simulink model "linearization"  (Simulink 8.7)
settings: Solver=VariableStepAuto  StartTime=0.0  StopTime=10.0  RelTol=1e-3
undefined symbols (not defined in the file or in its folder): CONFIG, DiscIntNeverNeededParam, gain, reg, ROBOT_DOF, ROBOT_DOF_FOR_SIMULINK, WBT_robotName
libraries: WBToolboxLibrary x42
settings Model: Creator=gnava  LastModifiedBy=gnava
settings DataIOCC: LimitDataPoints=off  SaveFormat=Dataset
settings DebuggingCC: UnderspecifiedInitializationDetection=Simplified  MergeDetectMultiDrivingBlocksExec=error
settings HardwareCC: ProdBitPerPointer=64  ProdLargestAtomicFloat=Float  ProdIntDivRoundTo=Zero  ProdEndianess=LittleEndian  ProdWordSize=64  ProdHWDeviceType=Intel->x86-64 (Windows64)
settings ModelReferenceCC: PropagateSignalLabelsOutOfModel=on
settings ConfigComp: CovModelRefEnable=off

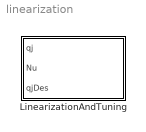
== system linearization ==
  LinearizationAndTuning : Subsystem

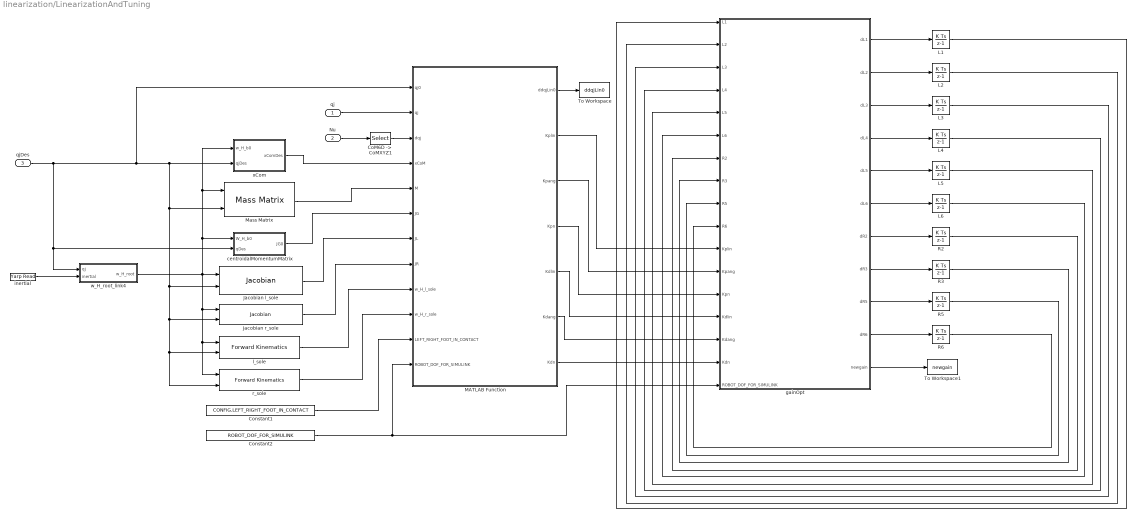
== system linearization/LinearizationAndTuning ==
  qj : Inport
  Nu : Inport  Port=2
  qjDes : Inport  Port=3
  "CoM6D ->  CoMXYZ1" : Selector  InputPortWidth=6+ROBOT_DOF  IndexOptions=Index vector (dialog)  Indices=[7:6+ROBOT_DOF]  OutputSizes=1
  Constant1 : Constant  Value=CONFIG.LEFT_RIGHT_FOOT_IN_CONTACT
  Constant2 : Constant  Value=ROBOT_DOF_FOR_SIMULINK
  Jacobian l_sole : WBToolboxLibrary/wholeBodyModel/Jacobians/Jacobian  frameName='l_sole'  robotName=WBT_robotName  localName=WBT_modelName  wbiFile=WBT_wbiFilename  wbiList=WBT_wbiList
  Jacobian r_sole : WBToolboxLibrary/wholeBodyModel/Jacobians/Jacobian  frameName='r_sole'  robotName=WBT_robotName  localName=WBT_modelName  wbiFile=WBT_wbiFilename  wbiList=WBT_wbiList
  L1 : DiscreteIntegrator  InitialCondition=gain.CI1  InitialConditionSetting=State (most efficient)  SampleTime=CONFIG.Ts  ICPrevOutput=DiscIntNeverNeededParam  ICPrevScaledInput=DiscIntNeverNeededParam
  L2 : DiscreteIntegrator  InitialCondition=gain.CI2  InitialConditionSetting=State (most efficient)  SampleTime=CONFIG.Ts  ICPrevOutput=DiscIntNeverNeededParam  ICPrevScaledInput=DiscIntNeverNeededParam
  L3 : DiscreteIntegrator  InitialCondition=gain.CI3  InitialConditionSetting=State (most efficient)  SampleTime=CONFIG.Ts  ICPrevOutput=DiscIntNeverNeededParam  ICPrevScaledInput=DiscIntNeverNeededParam
  L4 : DiscreteIntegrator  InitialCondition=gain.CI4  InitialConditionSetting=State (most efficient)  SampleTime=CONFIG.Ts  ICPrevOutput=DiscIntNeverNeededParam  ICPrevScaledInput=DiscIntNeverNeededParam
  L5 : DiscreteIntegrator  InitialCondition=gain.CI5  InitialConditionSetting=State (most efficient)  SampleTime=CONFIG.Ts  ICPrevOutput=DiscIntNeverNeededParam  ICPrevScaledInput=DiscIntNeverNeededParam
  L6 : DiscreteIntegrator  InitialCondition=gain.CI6  InitialConditionSetting=State (most efficient)  SampleTime=CONFIG.Ts  ICPrevOutput=DiscIntNeverNeededParam  ICPrevScaledInput=DiscIntNeverNeededParam
  MATLAB Function : MATLAB Function  TreatAsAtomicUnit=on
  Mass Matrix : WBToolboxLibrary/wholeBodyModel/Dynamics/Mass Matrix  robotName=WBT_robotName  localName=WBT_modelName  wbiFile=WBT_wbiFilename  wbiList=WBT_wbiList
  R2 : DiscreteIntegrator  InitialCondition=eye(3)  InitialConditionSetting=State (most efficient)  SampleTime=CONFIG.Ts  ICPrevOutput=DiscIntNeverNeededParam  ICPrevScaledInput=DiscIntNeverNeededParam
  R3 : DiscreteIntegrator  InitialCondition=eye(ROBOT_DOF)  InitialConditionSetting=State (most efficient)  SampleTime=CONFIG.Ts  ICPrevOutput=DiscIntNeverNeededParam  ICPrevScaledInput=DiscIntNeverNeededParam
  R5 : DiscreteIntegrator  InitialCondition=eye(3)  InitialConditionSetting=State (most efficient)  SampleTime=CONFIG.Ts  ICPrevOutput=DiscIntNeverNeededParam  ICPrevScaledInput=DiscIntNeverNeededParam
  R6 : DiscreteIntegrator  InitialCondition=eye(ROBOT_DOF)  InitialConditionSetting=State (most efficient)  SampleTime=CONFIG.Ts  ICPrevOutput=DiscIntNeverNeededParam  ICPrevScaledInput=DiscIntNeverNeededParam
  To Workspace : ToWorkspace  VariableName=ddqjLin0  SaveFormat=Structure With Time  SampleTime=-1
  To Workspace1 : ToWorkspace  VariableName=newgain  SaveFormat=Structure With Time  SampleTime=-1
  centroidalMomentumMatrix : Subsystem
  gainOpt : MATLAB Function  TreatAsAtomicUnit=on
  inertial : WBToolboxLibrary/Utilities/Yarp Read  portName=PORTS.IMU  signalSize=12  blocking=off  timestamp=off  autoconnect=on  errorOnConnection=on
  l_sole : WBToolboxLibrary/wholeBodyModel/Kinematics/Forward Kinematics  frameName='l_sole'  robotName=WBT_robotName  localName=WBT_modelName  wbiFile=WBT_wbiFilename  wbiList=WBT_wbiList
  r_sole : WBToolboxLibrary/wholeBodyModel/Kinematics/Forward Kinematics  frameName='r_sole'  robotName=WBT_robotName  localName=WBT_modelName  wbiFile=WBT_wbiFilename  wbiList=WBT_wbiList
  w_H_root_link4 : Subsystem  mask{link_name='l_sole'}
      mask prompts: link_name "link name"
      mask help:
      | This block evaluates the homogeneous transformation between the world and the root link, i.e. ^wH_b. It assumes that the link specified by the variable 'link_name' has a constant position
      | w.r.t. an inertial frame, but it can rotate arbitrarily. This rotation is retrived from the IMU sensor.
      mask Display:
      | str = strrep(link_name, '_','\_');
      | port_label('output',1,['{}^{',str '}H_{root}'],'texmode','on')
      | clear str;
      | 
      | port_label('input',1,'q_j','texmode','on')
      | 
      | port_label('input',2,'inertial','texmode','on')
  xCom : Subsystem
  wires:
  w_H_root_link4/1(w_H_root) -> xCom/1(w_H_b0), Mass Matrix/1, centroidalMomentumMatrix/1(W_H_b0), Jacobian l_sole/1, Jacobian r_sole/1, l_sole/1, r_sole/1
  inertial/1 -> w_H_root_link4/2(inertial)
  qjDes/1 -> Mass Matrix/2, Jacobian l_sole/2, Jacobian r_sole/2, l_sole/2, r_sole/2, xCom/2(qjDes), MATLAB Function/1(qj0), w_H_root_link4/1(qj), centroidalMomentumMatrix/2(qDes)
  xCom/1(xComDes) -> MATLAB Function/4(xCoM)
  Mass Matrix/1 -> MATLAB Function/5(M)
  Constant1/1 -> MATLAB Function/11(LEFT_RIGHT_FOOT_IN_CONTACT)
  Jacobian l_sole/1 -> MATLAB Function/7(JL)
  Jacobian r_sole/1 -> MATLAB Function/8(JR)
  l_sole/1 -> MATLAB Function/9(w_H_l_sole)
  r_sole/1 -> MATLAB Function/10(w_H_r_sole)
  centroidalMomentumMatrix/1(JG0) -> MATLAB Function/6(JG)
  Nu/1 -> "CoM6D ->  CoMXYZ1"/1
  qj/1 -> MATLAB Function/2(qj)
  "CoM6D ->  CoMXYZ1"/1 -> MATLAB Function/3(dqj)
  MATLAB Function/1(ddqjLin0) -> To Workspace/1
  Constant2/1 -> gainOpt/17(ROBOT_DOF_FOR_SIMULINK), MATLAB Function/12(ROBOT_DOF_FOR_SIMULINK)
  MATLAB Function/7(Kdn) -> gainOpt/16(Kdn)
  MATLAB Function/6(Kdang) -> gainOpt/15(Kdang)
  MATLAB Function/5(Kdlin) -> gainOpt/14(Kdlin)
  MATLAB Function/4(Kpn) -> gainOpt/13(Kpn)
  MATLAB Function/3(Kpang) -> gainOpt/12(Kpang)
  MATLAB Function/2(Kplin) -> gainOpt/11(Kplin)
  gainOpt/11(newgain) -> To Workspace1/1
  gainOpt/1(dL1) -> L1/1
  gainOpt/2(dL2) -> L2/1
  gainOpt/3(dL3) -> L3/1
  gainOpt/4(dL4) -> L4/1
  gainOpt/5(dL5) -> L5/1
  gainOpt/6(dL6) -> L6/1
  gainOpt/7(dR2) -> R2/1
  gainOpt/8(dR3) -> R3/1
  gainOpt/9(dR5) -> R5/1
  gainOpt/10(dR6) -> R6/1
  L1/1 -> gainOpt/1(L1)
  L2/1 -> gainOpt/2(L2)
  L3/1 -> gainOpt/3(L3)
  L4/1 -> gainOpt/4(L4)
  L5/1 -> gainOpt/5(L5)
  L6/1 -> gainOpt/6(L6)
  R2/1 -> gainOpt/7(R2)
  R3/1 -> gainOpt/8(R3)
  R5/1 -> gainOpt/9(R5)
  R6/1 -> gainOpt/10(R6)

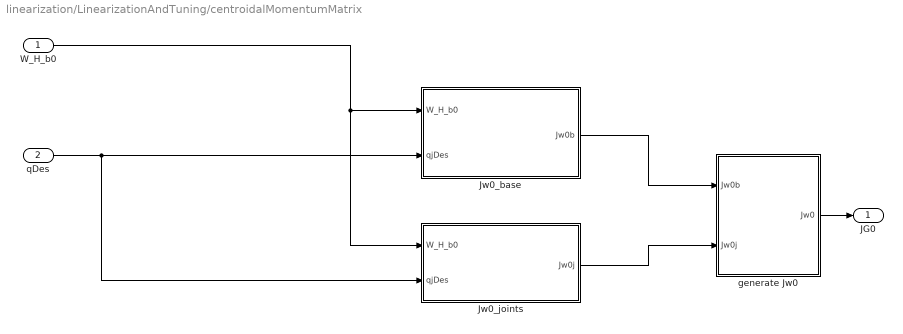
== system linearization/LinearizationAndTuning/centroidalMomentumMatrix ==
  W_H_b0 : Inport
  qDes : Inport  Port=2
  Jw0_base : Subsystem
  Jw0_joints : Subsystem
  generate Jw0 : MATLAB Function  TreatAsAtomicUnit=on
  JG0 : Outport
  wires:
  generate Jw0/1(Jw0) -> JG0/1
  W_H_b0/1 -> Jw0_joints/1(W_H_b0), Jw0_base/1(W_H_b0)
  qDes/1 -> Jw0_base/2(qjDes), Jw0_joints/2(qjDes)
  Jw0_base/1(Jw0b) -> generate Jw0/1(Jw0b)
  Jw0_joints/1(Jw0j) -> generate Jw0/2(Jw0j)

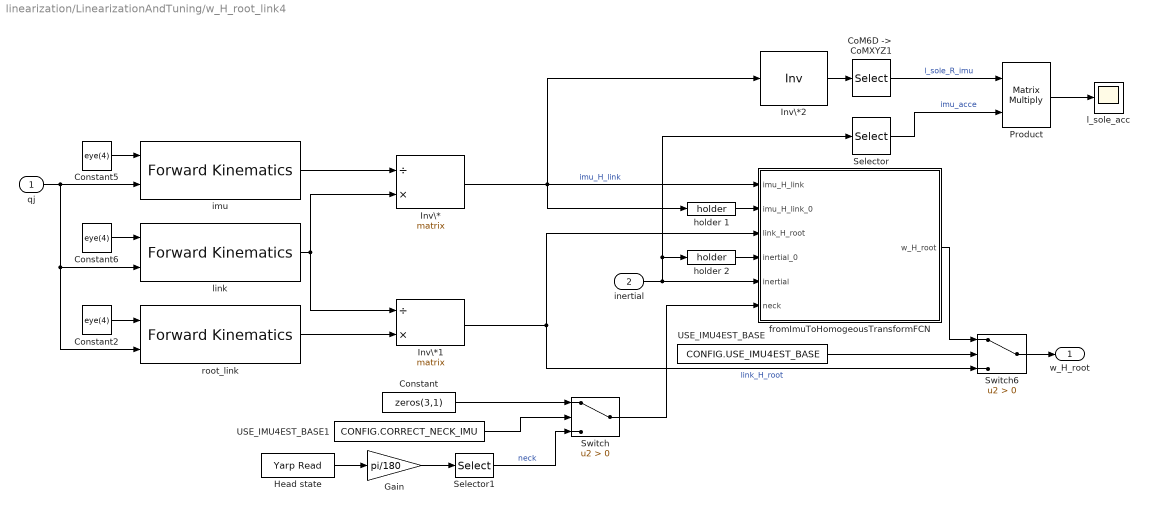
== system linearization/LinearizationAndTuning/w_H_root_link4 ==
  qj : Inport
  inertial : Inport  Port=2
  "CoM6D ->  CoMXYZ1" : Selector  NumberOfDimensions=2  InputPortWidth=7  IndexOptions=Index vector (dialog),Index vector (dialog)  Indices=[1 2 3],[1 2 3]  OutputSizes=1,1
  Constant : Constant  Value=zeros(3,1)
  Constant2 : Constant  Value=eye(4)
  Constant5 : Constant  Value=eye(4)
  Constant6 : Constant  Value=eye(4)
  Gain : Gain  Gain=pi/180
  Head state : WBToolboxLibrary/Utilities/Yarp Read  portName=[WBT_robotName, '/head/state:o']  signalSize=6  blocking=off  timestamp=off  autoconnect=on  errorOnConnection=off
  Inv\* : Product  Inputs=/*  Multiplication=Matrix(*)
  Inv\*1 : Product  Inputs=/*  Multiplication=Matrix(*)
  Inv\*2 : Product  Inputs=/  Multiplication=Matrix(*)
  Product : Product  Multiplication=Matrix(*)
  Selector : Selector  InputPortWidth=12  IndexOptions=Index vector (dialog)  Indices=[4 5 6 ]  OutputSizes=1
  Selector1 : Selector  InputPortWidth=6  IndexOptions=Index vector (dialog)  Indices=[1:3]  OutputSizes=1
  Switch : Switch  Criteria=u2 > Threshold
  Switch6 : Switch  Criteria=u2 > Threshold
  USE_IMU4EST_BASE : Constant  Value=CONFIG.USE_IMU4EST_BASE
  USE_IMU4EST_BASE1 : Constant  Value=CONFIG.CORRECT_NECK_IMU
  fromImuToHomogeousTransformFCN : MATLAB Function  TreatAsAtomicUnit=on
  holder 1 : WBToolboxLibrary/Utilities/holder 
  holder 2 : WBToolboxLibrary/Utilities/holder 
  imu : WBToolboxLibrary/wholeBodyModel/Kinematics/Forward Kinematics  frameName='imu_frame'  robotName=WBT_robotName  localName=WBT_modelName  wbiFile=WBT_wbiFilename  wbiList=WBT_wbiList
  l_sole_acc : Scope
  link : WBToolboxLibrary/wholeBodyModel/Kinematics/Forward Kinematics  frameName=link_name  robotName=WBT_robotName  localName=WBT_modelName  wbiFile=WBT_wbiFilename  wbiList=WBT_wbiList
  root_link : WBToolboxLibrary/wholeBodyModel/Kinematics/Forward Kinematics  frameName='root_link'  robotName=WBT_robotName  localName=WBT_modelName  wbiFile=WBT_wbiFilename  wbiList=WBT_wbiList
  w_H_root : Outport
  wires:
  Constant5/1 -> imu/1
  Inv\*/1 -> Inv\*2/1, holder 1/1, fromImuToHomogeousTransformFCN/1(imu_H_link)  "imu_H_link"
  imu/1 -> Inv\*/1
  Constant6/1 -> link/1
  Inv\*1/1 -> Switch6/3, fromImuToHomogeousTransformFCN/3(link_H_root)  "link_H_root"
  link/1 -> Inv\*/2, Inv\*1/1
  inertial/1 -> Selector/1, holder 2/1, fromImuToHomogeousTransformFCN/5(inertial)
  Switch6/1 -> w_H_root/1
  USE_IMU4EST_BASE/1 -> Switch6/2
  fromImuToHomogeousTransformFCN/1(w_H_root) -> Switch6/1
  Constant2/1 -> root_link/1
  qj/1 -> root_link/2, link/2, imu/2
  root_link/1 -> Inv\*1/2
  holder 1/1 -> fromImuToHomogeousTransformFCN/2(imu_H_link_0)
  holder 2/1 -> fromImuToHomogeousTransformFCN/4(inertial_0)
  Inv\*2/1 -> "CoM6D ->  CoMXYZ1"/1
  "CoM6D ->  CoMXYZ1"/1 -> Product/1  "l_sole_R_imu"
  Selector/1 -> Product/2  "imu_acce"
  Product/1 -> l_sole_acc/1
  Head state/1 -> Gain/1
  Selector1/1 -> Switch/3  "neck"
  Constant/1 -> Switch/1
  USE_IMU4EST_BASE1/1 -> Switch/2
  Switch/1 -> fromImuToHomogeousTransformFCN/6(neck)
  Gain/1 -> Selector1/1

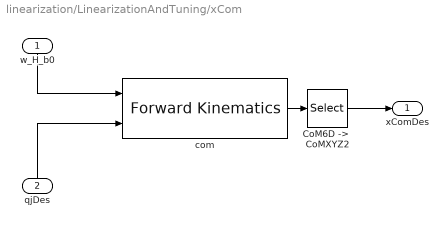
== system linearization/LinearizationAndTuning/xCom ==
  w_H_b0 : Inport
  qjDes : Inport  Port=2
  "CoM6D ->  CoMXYZ2" : Selector  NumberOfDimensions=2  InputPortWidth=7  IndexOptions=Index vector (dialog),Index vector (dialog)  Indices=[1 2 3],[4]  OutputSizes=1,1
  com : WBToolboxLibrary/wholeBodyModel/Kinematics/Forward Kinematics  frameName='com'  robotName=WBT_robotName  localName=WBT_modelName  wbiFile=WBT_wbiFilename  wbiList=WBT_wbiList
  xComDes : Outport
  wires:
  qjDes/1 -> com/2
  "CoM6D ->  CoMXYZ2"/1 -> xComDes/1
  com/1 -> "CoM6D ->  CoMXYZ2"/1
  w_H_b0/1 -> com/1

== system linearization/LinearizationAndTuning/centroidalMomentumMatrix/Jw0_base ==
  W_H_b0 : Inport
  qjDes : Inport  Port=2
  Generate_Jw0base : Subsystem
  Jw0b : Outport
  wires:
  Generate_Jw0base/1(Jw0b) -> Jw0b/1
  qjDes/1 -> Generate_Jw0base/1(qjDes)
  W_H_b0/1 -> Generate_Jw0base/2(W_H_B0)

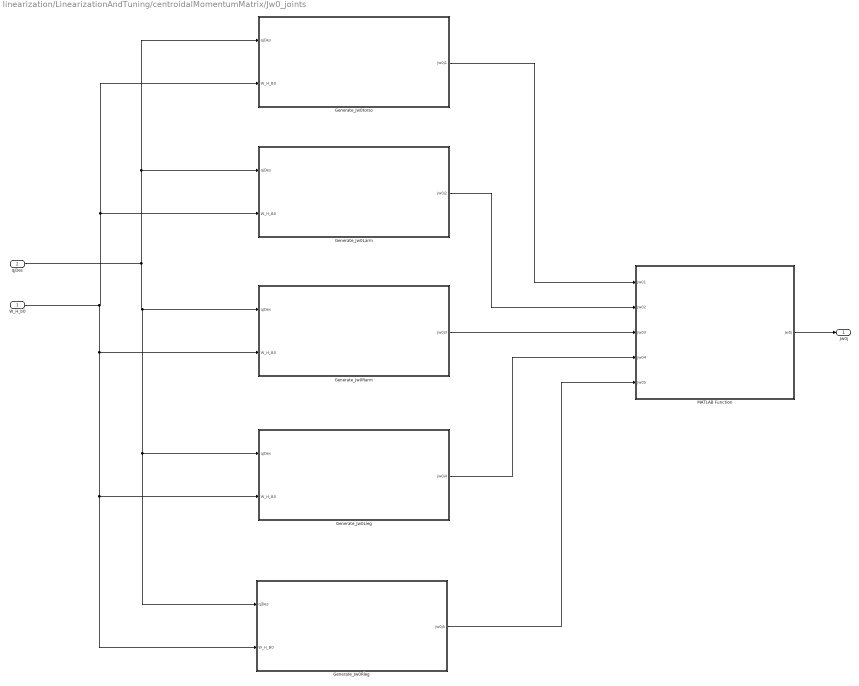
== system linearization/LinearizationAndTuning/centroidalMomentumMatrix/Jw0_joints ==
  W_H_b0 : Inport
  qjDes : Inport  Port=2
  Generate_Jw0Larm : Subsystem
  Generate_Jw0Lleg : Subsystem
  Generate_Jw0Rarm : Subsystem
  Generate_Jw0Rleg : Subsystem
  Generate_Jw0torso : Subsystem
  MATLAB Function : MATLAB Function  TreatAsAtomicUnit=on
  Jw0j : Outport
  wires:
  qjDes/1 -> Generate_Jw0Rarm/1(qjDes), Generate_Jw0Rleg/1(qjDes), Generate_Jw0Lleg/1(qjDes), Generate_Jw0Larm/1(qjDes), Generate_Jw0torso/1(qjDes)
  W_H_b0/1 -> Generate_Jw0Rarm/2(W_H_B0), Generate_Jw0Rleg/2(W_H_B0), Generate_Jw0Lleg/2(W_H_B0), Generate_Jw0Larm/2(W_H_B0), Generate_Jw0torso/2(W_H_B0)
  Generate_Jw0torso/1(Jw0j1) -> MATLAB Function/1(Jw01)
  Generate_Jw0Larm/1(Jw0j2) -> MATLAB Function/2(Jw02)
  Generate_Jw0Rarm/1(Jw0j3) -> MATLAB Function/3(Jw03)
  Generate_Jw0Lleg/1(Jw0j4) -> MATLAB Function/4(Jw04)
  Generate_Jw0Rleg/1(Jw0j5) -> MATLAB Function/5(Jw05)
  MATLAB Function/1(Jw0j) -> Jw0j/1

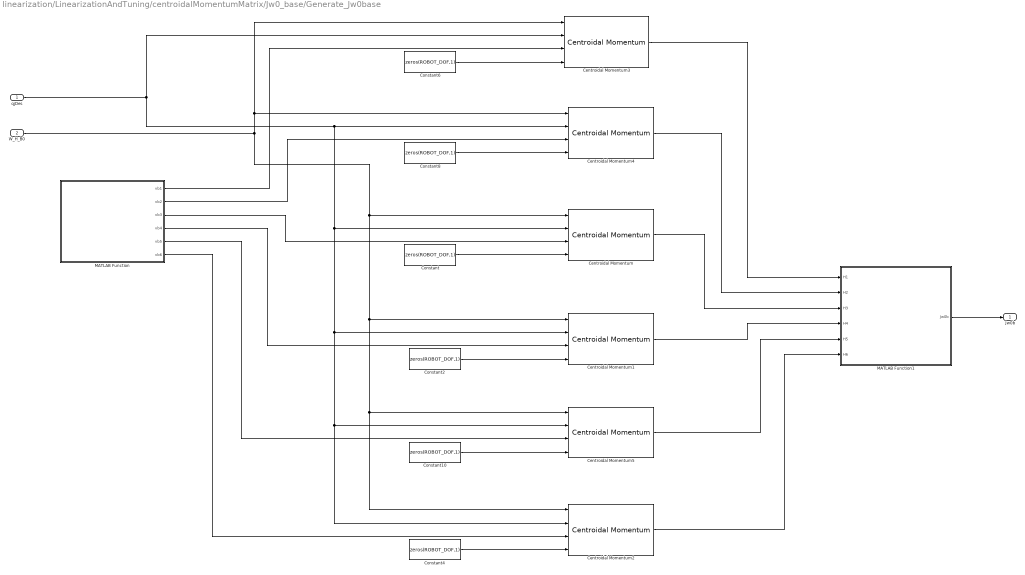
== system linearization/LinearizationAndTuning/centroidalMomentumMatrix/Jw0_base/Generate_Jw0base ==
  qjDes : Inport
  W_H_B0 : Inport  Port=2
  Centroidal Momentum{,1..5} (6 alike) : WBToolboxLibrary/wholeBodyModel/Dynamics/Centroidal Momentum  robotName=WBT_robotName  localName=WBT_modelName  wbiFile=WBT_wbiFilename  wbiList=WBT_wbiList
  Constant{,2,4,6,8,10} (6 alike) : Constant  Value=zeros(ROBOT_DOF,1)
  MATLAB Function : MATLAB Function  TreatAsAtomicUnit=on
  MATLAB Function1 : MATLAB Function  TreatAsAtomicUnit=on
  Jw0b : Outport
  wires:
  MATLAB Function/1(vb1) -> Centroidal Momentum3/3
  MATLAB Function/2(vb2) -> Centroidal Momentum4/3
  MATLAB Function/3(vb3) -> Centroidal Momentum/3
  MATLAB Function/4(vb4) -> Centroidal Momentum1/3
  MATLAB Function/5(vb5) -> Centroidal Momentum5/3
  MATLAB Function/6(vb6) -> Centroidal Momentum2/3
  Constant6/1 -> Centroidal Momentum3/4
  Constant8/1 -> Centroidal Momentum4/4
  Constant/1 -> Centroidal Momentum/4
  Constant2/1 -> Centroidal Momentum1/4
  Constant10/1 -> Centroidal Momentum5/4
  Constant4/1 -> Centroidal Momentum2/4
  qjDes/1 -> Centroidal Momentum2/2, Centroidal Momentum5/2, Centroidal Momentum1/2, Centroidal Momentum/2, Centroidal Momentum4/2, Centroidal Momentum3/2
  W_H_B0/1 -> Centroidal Momentum3/1, Centroidal Momentum4/1, Centroidal Momentum2/1, Centroidal Momentum5/1, Centroidal Momentum1/1, Centroidal Momentum/1
  Centroidal Momentum3/1 -> MATLAB Function1/1(H1)
  Centroidal Momentum4/1 -> MATLAB Function1/2(H2)
  Centroidal Momentum/1 -> MATLAB Function1/3(H3)
  Centroidal Momentum1/1 -> MATLAB Function1/4(H4)
  Centroidal Momentum5/1 -> MATLAB Function1/5(H5)
  Centroidal Momentum2/1 -> MATLAB Function1/6(H6)
  MATLAB Function1/1(Jw0b) -> Jw0b/1

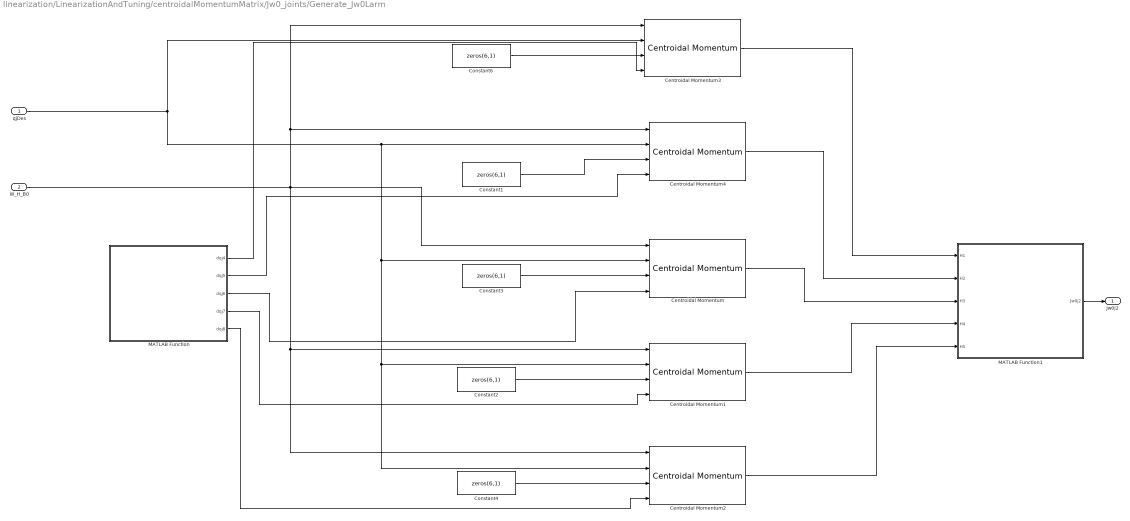
== system linearization/LinearizationAndTuning/centroidalMomentumMatrix/Jw0_joints/Generate_Jw0Larm ==
  qjDes : Inport
  W_H_B0 : Inport  Port=2
  Centroidal Momentum{,1..4} (5 alike) : WBToolboxLibrary/wholeBodyModel/Dynamics/Centroidal Momentum  robotName=WBT_robotName  localName=WBT_modelName  wbiFile=WBT_wbiFilename  wbiList=WBT_wbiList
  Constant{1..4,6} (5 alike) : Constant  Value=zeros(6,1)
  MATLAB Function : MATLAB Function  TreatAsAtomicUnit=on
  MATLAB Function1 : MATLAB Function  TreatAsAtomicUnit=on
  Jw0j2 : Outport
  wires:
  qjDes/1 -> Centroidal Momentum2/2, Centroidal Momentum1/2, Centroidal Momentum/2, Centroidal Momentum4/2, Centroidal Momentum3/2
  W_H_B0/1 -> Centroidal Momentum3/1, Centroidal Momentum4/1, Centroidal Momentum2/1, Centroidal Momentum1/1, Centroidal Momentum/1
  Centroidal Momentum3/1 -> MATLAB Function1/1(H1)
  Centroidal Momentum4/1 -> MATLAB Function1/2(H2)
  Centroidal Momentum/1 -> MATLAB Function1/3(H3)
  MATLAB Function1/1(Jw0j2) -> Jw0j2/1
  Constant6/1 -> Centroidal Momentum3/3
  Constant1/1 -> Centroidal Momentum4/3
  Constant3/1 -> Centroidal Momentum/3
  Constant4/1 -> Centroidal Momentum2/3
  Constant2/1 -> Centroidal Momentum1/3
  Centroidal Momentum1/1 -> MATLAB Function1/4(H4)
  Centroidal Momentum2/1 -> MATLAB Function1/5(H5)
  MATLAB Function/1(dqj4) -> Centroidal Momentum3/4
  MATLAB Function/2(dqj5) -> Centroidal Momentum4/4
  MATLAB Function/3(dqj6) -> Centroidal Momentum/4
  MATLAB Function/4(dqj7) -> Centroidal Momentum1/4
  MATLAB Function/5(dqj8) -> Centroidal Momentum2/4

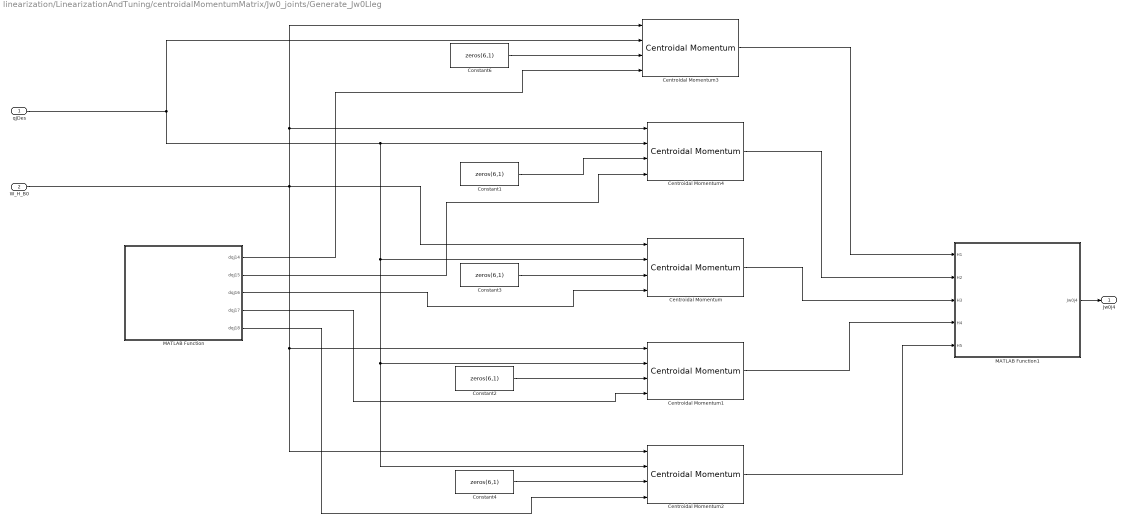
== system linearization/LinearizationAndTuning/centroidalMomentumMatrix/Jw0_joints/Generate_Jw0Lleg ==
  qjDes : Inport
  W_H_B0 : Inport  Port=2
  Centroidal Momentum{,1..4} (5 alike) : WBToolboxLibrary/wholeBodyModel/Dynamics/Centroidal Momentum  robotName=WBT_robotName  localName=WBT_modelName  wbiFile=WBT_wbiFilename  wbiList=WBT_wbiList
  Constant{1..4,6} (5 alike) : Constant  Value=zeros(6,1)
  MATLAB Function : MATLAB Function  TreatAsAtomicUnit=on
  MATLAB Function1 : MATLAB Function  TreatAsAtomicUnit=on
  Jw0j4 : Outport
  wires:
  qjDes/1 -> Centroidal Momentum2/2, Centroidal Momentum1/2, Centroidal Momentum/2, Centroidal Momentum4/2, Centroidal Momentum3/2
  W_H_B0/1 -> Centroidal Momentum3/1, Centroidal Momentum4/1, Centroidal Momentum2/1, Centroidal Momentum1/1, Centroidal Momentum/1
  Centroidal Momentum3/1 -> MATLAB Function1/1(H1)
  Centroidal Momentum4/1 -> MATLAB Function1/2(H2)
  Centroidal Momentum/1 -> MATLAB Function1/3(H3)
  MATLAB Function1/1(Jw0j4) -> Jw0j4/1
  Constant6/1 -> Centroidal Momentum3/3
  Constant1/1 -> Centroidal Momentum4/3
  Constant3/1 -> Centroidal Momentum/3
  MATLAB Function/1(dqj14) -> Centroidal Momentum3/4
  MATLAB Function/3(dqj16) -> Centroidal Momentum/4
  MATLAB Function/2(dqj15) -> Centroidal Momentum4/4
  Constant4/1 -> Centroidal Momentum2/3
  Constant2/1 -> Centroidal Momentum1/3
  Centroidal Momentum1/1 -> MATLAB Function1/4(H4)
  Centroidal Momentum2/1 -> MATLAB Function1/5(H5)
  MATLAB Function/4(dqj17) -> Centroidal Momentum1/4
  MATLAB Function/5(dqj18) -> Centroidal Momentum2/4

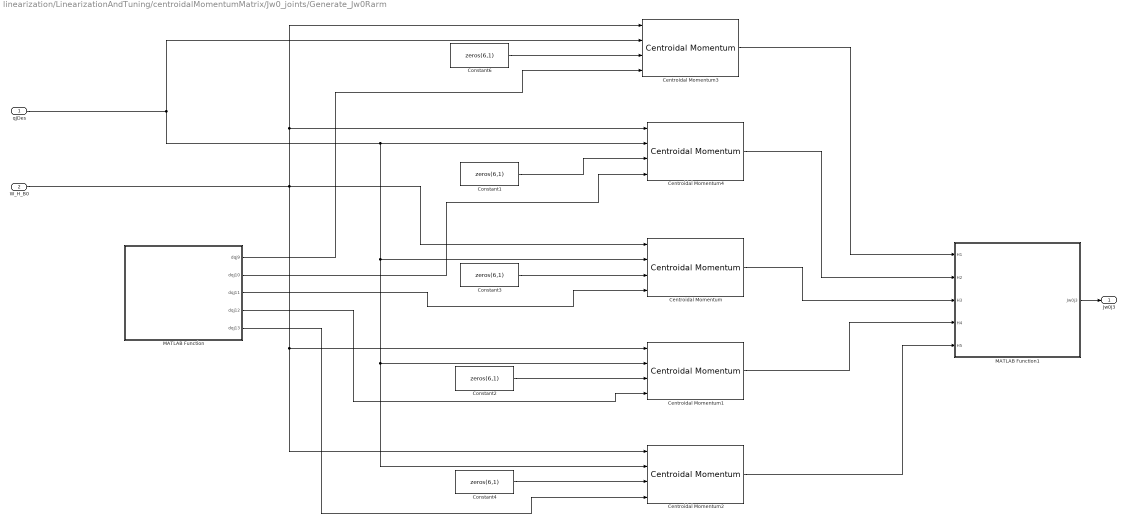
== system linearization/LinearizationAndTuning/centroidalMomentumMatrix/Jw0_joints/Generate_Jw0Rarm ==
  qjDes : Inport
  W_H_B0 : Inport  Port=2
  Centroidal Momentum{,1..4} (5 alike) : WBToolboxLibrary/wholeBodyModel/Dynamics/Centroidal Momentum  robotName=WBT_robotName  localName=WBT_modelName  wbiFile=WBT_wbiFilename  wbiList=WBT_wbiList
  Constant{1..4,6} (5 alike) : Constant  Value=zeros(6,1)
  MATLAB Function : MATLAB Function  TreatAsAtomicUnit=on
  MATLAB Function1 : MATLAB Function  TreatAsAtomicUnit=on
  Jw0j3 : Outport
  wires:
  qjDes/1 -> Centroidal Momentum2/2, Centroidal Momentum1/2, Centroidal Momentum/2, Centroidal Momentum4/2, Centroidal Momentum3/2
  W_H_B0/1 -> Centroidal Momentum3/1, Centroidal Momentum4/1, Centroidal Momentum2/1, Centroidal Momentum1/1, Centroidal Momentum/1
  Centroidal Momentum3/1 -> MATLAB Function1/1(H1)
  Centroidal Momentum4/1 -> MATLAB Function1/2(H2)
  Centroidal Momentum/1 -> MATLAB Function1/3(H3)
  MATLAB Function1/1(Jw0j3) -> Jw0j3/1
  Constant6/1 -> Centroidal Momentum3/3
  Constant1/1 -> Centroidal Momentum4/3
  Constant3/1 -> Centroidal Momentum/3
  MATLAB Function/1(dqj9) -> Centroidal Momentum3/4
  MATLAB Function/3(dqj11) -> Centroidal Momentum/4
  MATLAB Function/2(dqj10) -> Centroidal Momentum4/4
  Constant4/1 -> Centroidal Momentum2/3
  Constant2/1 -> Centroidal Momentum1/3
  Centroidal Momentum1/1 -> MATLAB Function1/4(H4)
  Centroidal Momentum2/1 -> MATLAB Function1/5(H5)
  MATLAB Function/4(dqj12) -> Centroidal Momentum1/4
  MATLAB Function/5(dqj13) -> Centroidal Momentum2/4

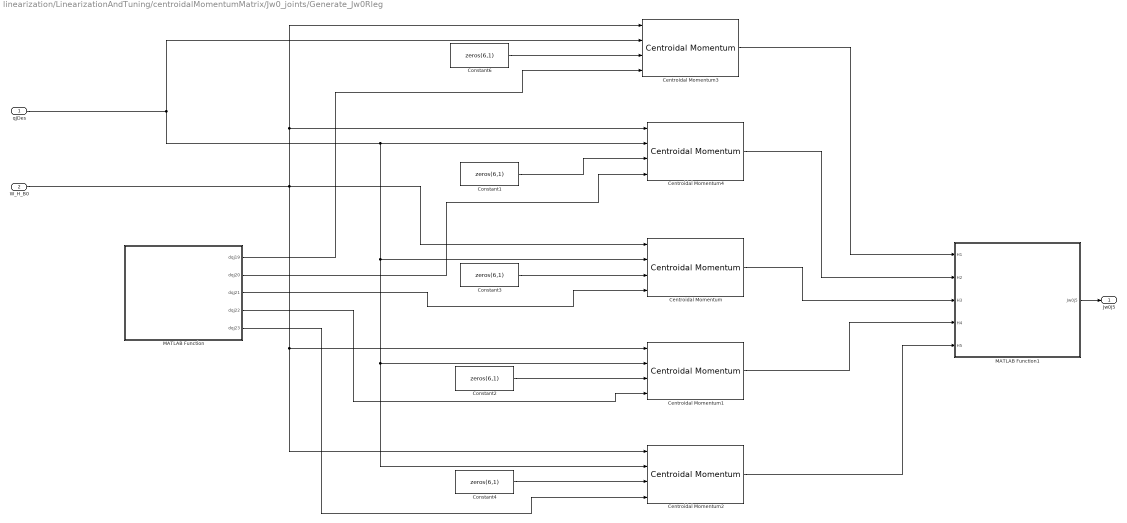
== system linearization/LinearizationAndTuning/centroidalMomentumMatrix/Jw0_joints/Generate_Jw0Rleg ==
  qjDes : Inport
  W_H_B0 : Inport  Port=2
  Centroidal Momentum{,1..4} (5 alike) : WBToolboxLibrary/wholeBodyModel/Dynamics/Centroidal Momentum  robotName=WBT_robotName  localName=WBT_modelName  wbiFile=WBT_wbiFilename  wbiList=WBT_wbiList
  Constant{1..4,6} (5 alike) : Constant  Value=zeros(6,1)
  MATLAB Function : MATLAB Function  TreatAsAtomicUnit=on
  MATLAB Function1 : MATLAB Function  TreatAsAtomicUnit=on
  Jw0j5 : Outport
  wires:
  qjDes/1 -> Centroidal Momentum2/2, Centroidal Momentum1/2, Centroidal Momentum/2, Centroidal Momentum4/2, Centroidal Momentum3/2
  W_H_B0/1 -> Centroidal Momentum3/1, Centroidal Momentum4/1, Centroidal Momentum2/1, Centroidal Momentum1/1, Centroidal Momentum/1
  Centroidal Momentum3/1 -> MATLAB Function1/1(H1)
  Centroidal Momentum4/1 -> MATLAB Function1/2(H2)
  Centroidal Momentum/1 -> MATLAB Function1/3(H3)
  MATLAB Function1/1(Jw0j5) -> Jw0j5/1
  Constant6/1 -> Centroidal Momentum3/3
  Constant1/1 -> Centroidal Momentum4/3
  Constant3/1 -> Centroidal Momentum/3
  MATLAB Function/1(dqj19) -> Centroidal Momentum3/4
  MATLAB Function/3(dqj21) -> Centroidal Momentum/4
  MATLAB Function/2(dqj20) -> Centroidal Momentum4/4
  Constant4/1 -> Centroidal Momentum2/3
  Constant2/1 -> Centroidal Momentum1/3
  Centroidal Momentum1/1 -> MATLAB Function1/4(H4)
  Centroidal Momentum2/1 -> MATLAB Function1/5(H5)
  MATLAB Function/4(dqj22) -> Centroidal Momentum1/4
  MATLAB Function/5(dqj23) -> Centroidal Momentum2/4

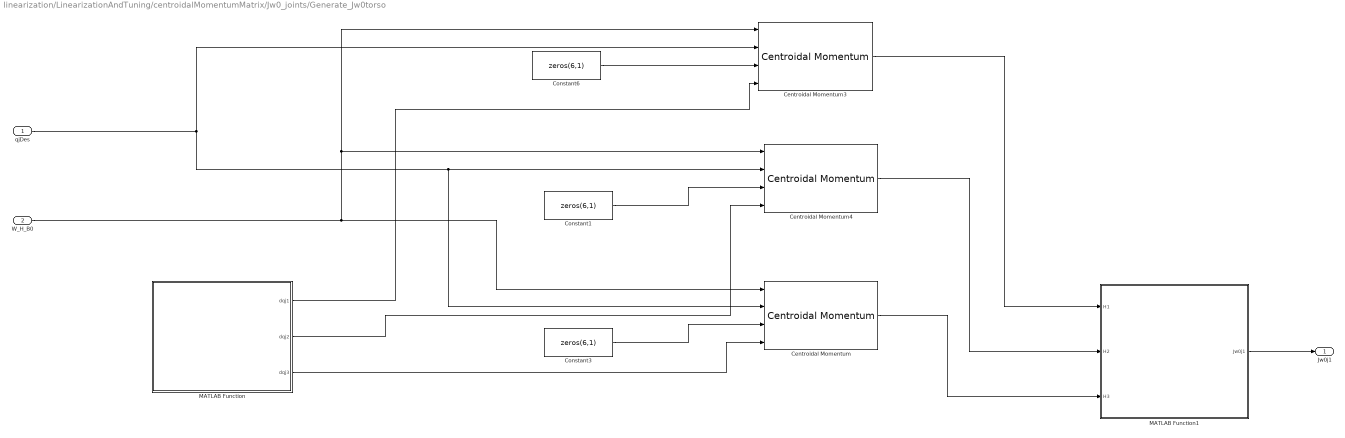
== system linearization/LinearizationAndTuning/centroidalMomentumMatrix/Jw0_joints/Generate_Jw0torso ==
  qjDes : Inport
  W_H_B0 : Inport  Port=2
  Centroidal Momentum : WBToolboxLibrary/wholeBodyModel/Dynamics/Centroidal Momentum  robotName=WBT_robotName  localName=WBT_modelName  wbiFile=WBT_wbiFilename  wbiList=WBT_wbiList
  Centroidal Momentum3 : WBToolboxLibrary/wholeBodyModel/Dynamics/Centroidal Momentum  robotName=WBT_robotName  localName=WBT_modelName  wbiFile=WBT_wbiFilename  wbiList=WBT_wbiList
  Centroidal Momentum4 : WBToolboxLibrary/wholeBodyModel/Dynamics/Centroidal Momentum  robotName=WBT_robotName  localName=WBT_modelName  wbiFile=WBT_wbiFilename  wbiList=WBT_wbiList
  Constant1 : Constant  Value=zeros(6,1)
  Constant3 : Constant  Value=zeros(6,1)
  Constant6 : Constant  Value=zeros(6,1)
  MATLAB Function : MATLAB Function  TreatAsAtomicUnit=on
  MATLAB Function1 : MATLAB Function  TreatAsAtomicUnit=on
  Jw0j1 : Outport
  wires:
  qjDes/1 -> Centroidal Momentum/2, Centroidal Momentum4/2, Centroidal Momentum3/2
  W_H_B0/1 -> Centroidal Momentum3/1, Centroidal Momentum4/1, Centroidal Momentum/1
  Centroidal Momentum3/1 -> MATLAB Function1/1(H1)
  Centroidal Momentum4/1 -> MATLAB Function1/2(H2)
  Centroidal Momentum/1 -> MATLAB Function1/3(H3)
  MATLAB Function1/1(Jw0j1) -> Jw0j1/1
  Constant6/1 -> Centroidal Momentum3/3
  Constant1/1 -> Centroidal Momentum4/3
  Constant3/1 -> Centroidal Momentum/3
  MATLAB Function/1(dqj1) -> Centroidal Momentum3/4
  MATLAB Function/3(dqj3) -> Centroidal Momentum/4
  MATLAB Function/2(dqj2) -> Centroidal Momentum4/4

== matlab function LinearizationAndTuning/gainOpt ==
  data: L1 input double; dL1 output double; dL2 output double; L2 input double; L3 input double; L4 input double; dL3 output double; dL4 output double; dL5 output double; dL6 output double; dR2 output double; L5 input double; L6 input double; R2 input double; R3 input double; R5 input double; R6 input double; Kplin input double; Kpang input double; Kpn input double; Kdlin input double; Kdang input double; Kdn input double; ROBOT_DOF_FOR_SIMULINK input double; dR3 output double; dR5 output double; dR6 output double; newgain output double
function [dL1,dL2,dL3,dL4,dL5,dL6,dR2,dR3,dR5,dR6,newgain] = optimizer(L1,L2,L3,L4,L5,L6,R2,R3,R5,R6,....
                                                                       Kplin,Kpang,Kpn,Kdlin,Kdang,Kdn,ROBOT_DOF_FOR_SIMULINK)

%%
R1 = eye(3);
R4 = R1;

[dL1,~,Kplin]   = optimConstr(L1,R1,Kplin,ROBOT_DOF_FOR_SIMULINK);
[dL2,dR2,Kpang] = optimConstr(L2,R2,Kpang,ROBOT_DOF_FOR_SIMULINK);
[dL3,dR3,Kpn]   = optimConstr(L3,R3,Kpn,ROBOT_DOF_FOR_SIMULINK);
[dL4,~,Kdlin]   = optimConstr(L4,R4,Kdlin,ROBOT_DOF_FOR_SIMULINK);
[dL5,dR5,Kdang] = optimConstr(L5,R5,Kdang,ROBOT_DOF_FOR_SIMULINK);
[dL6,dR6,Kdn]   = optimConstr(L6,R6,Kdn,ROBOT_DOF_FOR_SIMULINK);


newgain.Kplin = Kplin;
newgain.Kpang = Kpang;
newgain.Kpn   = Kpn;
newgain.Kdlin = Kdlin;
newgain.Kdang = Kdang;
newgain.Kdn   = Kdn;

== matlab function LinearizationAndTuning/MATLAB Function ==
  data: qj0 input double; qj input double; dqj input double; xCoM input double; ddqjLin0 output double; M input double; JG input double; JL input double; JR input double; w_H_l_sole input double; w_H_r_sole input double; LEFT_RIGHT_FOOT_IN_CONTACT input double; gain parameter double; reg parameter double; ROBOT_DOF_FOR_SIMULINK input double; Kplin output double; Kpang output double; Kpn output double; Kdlin output double; Kdang output double; Kdn output double
function [ddqjLin0,Kplin,Kpang,Kpn,Kdlin,Kdang,Kdn] = gainsTuningFCN(qj0,qj,dqj,xCoM,M,JG,JL,JR,w_H_l_sole,w_H_r_sole,...
                                                                     LEFT_RIGHT_FOOT_IN_CONTACT,gain,reg,ROBOT_DOF_FOR_SIMULINK) 
%#codegen
Jc = [LEFT_RIGHT_FOOT_IN_CONTACT(1)*JL;
      LEFT_RIGHT_FOOT_IN_CONTACT(2)*JR];

[KS,KD,Kplin,Kpang,Kpn,Kdlin,Kdang,Kdn]   = gainsTuning(xCoM,M,JG,Jc,w_H_l_sole,w_H_r_sole,LEFT_RIGHT_FOOT_IN_CONTACT,gain,reg,ROBOT_DOF_FOR_SIMULINK); 

ddqjLin0  = -KS*(qj-qj0)-KD*dqj;

== matlab function LinearizationAndTuning/w_H_root_link4/fromImuToHomogeousTransformFCN ==
  data: imu_H_link input double; imu_H_link_0 input double; link_H_root input double; inertial_0 input double; inertial input double; neck input double; w_H_root output double; CONFIG parameter double
function w_H_root = fromBaseToWorldWithImuFCN(imu_H_link,imu_H_link_0,link_H_root,inertial_0,inertial,neck,CONFIG)
%#codegen
w_H_root = fromBaseToWorldWithImu(imu_H_link,imu_H_link_0,link_H_root,inertial_0,inertial,neck,CONFIG);

== matlab function LinearizationAndTuning/centroidalMomentumMatrix/Jw0_base/Generate_Jw0base/MATLAB Function ==
  data: vb1 output double; vb2 output double; vb3 output double; vb4 output double; vb5 output double; vb6 output double
function [vb1,vb2, vb3, vb4, vb5, vb6] = gen_vb()
%#codegen

vb1 = [1;0;0;0;0;0];
vb2 = [0;1;0;0;0;0];
vb3 = [0;0;1;0;0;0];
vb4 = [0;0;0;1;0;0];
vb5 = [0;0;0;0;1;0];
vb6 = [0;0;0;0;0;1];

end

== matlab function LinearizationAndTuning/centroidalMomentumMatrix/Jw0_base/Generate_Jw0base/MATLAB Function1 ==
  data: H1 input double; Jw0b output double; H2 input double; H3 input double; H4 input double; H5 input double; H6 input double
function Jw0b = reorder_Jwb(H1,H2,H3,H4,H5,H6)
%#codegen

Jw0b = [H1 H2 H3 H4 H5 H6];

end

== matlab function LinearizationAndTuning/centroidalMomentumMatrix/Jw0_joints/Generate_Jw0Larm/MATLAB Function ==
  data: dqj4 output double; dqj5 output double; dqj6 output double; dqj7 output double; dqj8 output double
function [dqj4,dqj5, dqj6, dqj7, dqj8] = gen_vb()
%#codegen
ndof = 23;

dqj4 = zeros(ndof,1);
dqj5 = dqj4;
dqj6 = dqj5;
dqj7 = dqj6;
dqj8 = dqj7;

dqj4(4) = 1;
dqj5(5) = 1;
dqj6(6) = 1;
dqj7(7) = 1;
dqj8(8) = 1;

end

== matlab function LinearizationAndTuning/centroidalMomentumMatrix/Jw0_joints/Generate_Jw0Larm/MATLAB Function1 ==
  data: H1 input double; Jw0j2 output double; H2 input double; H3 input double; H4 input double; H5 input double
function Jw0j2 = reorder_Jwj(H1,H2,H3,H4,H5)
%#codegen

Jw0j2 = [H1 H2 H3 H4 H5];

end

== matlab function LinearizationAndTuning/centroidalMomentumMatrix/Jw0_joints/Generate_Jw0Lleg/MATLAB Function ==
  data: dqj14 output double; dqj15 output double; dqj16 output double; dqj17 output double; dqj18 output double
function [dqj14,dqj15, dqj16, dqj17, dqj18] = gen_vb()
%#codegen
ndof = 23;

dqj14 = zeros(ndof,1);
dqj15 = dqj14;
dqj16 = dqj15;
dqj17 = dqj16;
dqj18 = dqj17;

dqj14(14) = 1;
dqj15(15) = 1;
dqj16(16) = 1;
dqj17(17) = 1;
dqj18(18) = 1;

end

== matlab function LinearizationAndTuning/centroidalMomentumMatrix/Jw0_joints/Generate_Jw0Lleg/MATLAB Function1 ==
  data: H1 input double; Jw0j4 output double; H2 input double; H3 input double; H4 input double; H5 input double
function Jw0j4 = reorder_Jwj(H1,H2,H3,H4,H5)
%#codegen

Jw0j4 = [H1 H2 H3 H4 H5];

end

== matlab function LinearizationAndTuning/centroidalMomentumMatrix/Jw0_joints/Generate_Jw0Rarm/MATLAB Function ==
  data: dqj9 output double; dqj10 output double; dqj11 output double; dqj12 output double; dqj13 output double
function [dqj9,dqj10, dqj11, dqj12, dqj13] = gen_vb()
%#codegen
ndof = 23;

dqj9  = zeros(ndof,1);
dqj10 = dqj9;
dqj11 = dqj10;
dqj12 = dqj11;
dqj13 = dqj12;

dqj9(9)  = 1;
dqj10(10) = 1;
dqj11(11) = 1;
dqj12(12) = 1;
dqj13(13) = 1;

end

== matlab function LinearizationAndTuning/centroidalMomentumMatrix/Jw0_joints/Generate_Jw0Rarm/MATLAB Function1 ==
  data: H1 input double; Jw0j3 output double; H2 input double; H3 input double; H4 input double; H5 input double
function Jw0j3 = reorder_Jwj(H1,H2,H3,H4,H5)
%#codegen

Jw0j3 = [H1 H2 H3 H4 H5];

end

== matlab function LinearizationAndTuning/centroidalMomentumMatrix/Jw0_joints/Generate_Jw0Rleg/MATLAB Function ==
  data: dqj19 output double; dqj20 output double; dqj21 output double; dqj22 output double; dqj23 output double
function [dqj19,dqj20, dqj21, dqj22, dqj23] = gen_vb()
%#codegen
ndof = 23;

dqj19 = zeros(ndof,1);
dqj20 = dqj19;
dqj21 = dqj20;
dqj22 = dqj21;
dqj23 = dqj22;

dqj19(19) = 1;
dqj20(20) = 1;
dqj21(21) = 1;
dqj22(22) = 1;
dqj23(23) = 1;

end

== matlab function LinearizationAndTuning/centroidalMomentumMatrix/Jw0_joints/Generate_Jw0Rleg/MATLAB Function1 ==
  data: H1 input double; Jw0j5 output double; H2 input double; H3 input double; H4 input double; H5 input double
function Jw0j5 = reorder_Jwj(H1,H2,H3,H4,H5)
%#codegen

Jw0j5 = [H1 H2 H3 H4 H5];

end

== matlab function LinearizationAndTuning/centroidalMomentumMatrix/Jw0_joints/Generate_Jw0torso/MATLAB Function ==
  data: dqj1 output double; dqj2 output double; dqj3 output double
function [dqj1,dqj2,dqj3] = gen_vb()
%#codegen
ndof = 23;

dqj1 = zeros(ndof,1);
dqj2 = zeros(ndof,1);
dqj3 = zeros(ndof,1);

dqj1(1) = 1;
dqj2(2) = 1;
dqj3(3) = 1;

end

== matlab function LinearizationAndTuning/centroidalMomentumMatrix/Jw0_joints/Generate_Jw0torso/MATLAB Function1 ==
  data: H1 input double; Jw0j1 output double; H2 input double; H3 input double
function Jw0j1 = reorder_Jwj(H1,H2,H3)
%#codegen

Jw0j1 = [H1 H2 H3];

end

== matlab function LinearizationAndTuning/centroidalMomentumMatrix/Jw0_joints/MATLAB Function ==
  data: Jw01 input double; Jw0j output double; Jw02 input double; Jw03 input double; Jw04 input double; Jw05 input double
function Jw0j = fcn(Jw01,Jw02,Jw03,Jw04,Jw05)
%#codegen

Jw0j = [Jw01 Jw02 Jw03 Jw04 Jw05];

== matlab function LinearizationAndTuning/centroidalMomentumMatrix/generate Jw0 ==
  data: Jw0b input double; Jw0 output double; Jw0j input double
function Jw0 = generateJw0(Jw0b,Jw0j)
%#codegen

Jw0 = [Jw0b Jw0j];

end
